simulink model "q_aero_2dof_pid_control"  (R2014a)
settings: Solver=ode1  StartTime=0.0  StopTime=inf  FixedStep=0.002  RelTol=1e-3
PreLoadFcn:
  | quanser_aero_pd_design;
values from neighbouring files (symbols this model uses):
  kp_p = tau*wn^2/K    [quanser_aero_pd_design.m]    (also in quanser_aero_pd_design_Ksp.m = (Jp*wn^2-Ksp)/Kpp)
  kp_y = tau*wn^2/K    [quanser_aero_pd_design.m]    (also in quanser_aero_pd_design_Ksp.m = Jy*wn^2/Kyy)
libraries: simulink_extras x4, quarc_library x3, quanser_aero x1
settings Model: SimulationMode=external  ExtModeTrigDuration=15000  Creator=MLevis  LastModifiedBy=MLevis
settings SolverCC: PositivePriorityOrder=on
settings DebuggingCC: MergeDetectMultiDrivingBlocksExec=error
settings RTWCC: SystemTargetFile=quarc_win64.tlc  TemplateMakefile=quarc_default_tmf  Description=QUARC Win64 Target  ProcessScript=quarc_win64_make_rtw_hook
settings GRTTargetCC: ParMdlRefBuildCompliant=off  CompOptLevelCompliant=off  CombineOutputUpdateFcns=off  MatFileLogging=off  CPPClassGenCompliant=off  GRTInterface=on  ExtMode=on  ExtModeMexFile=quarc_comm

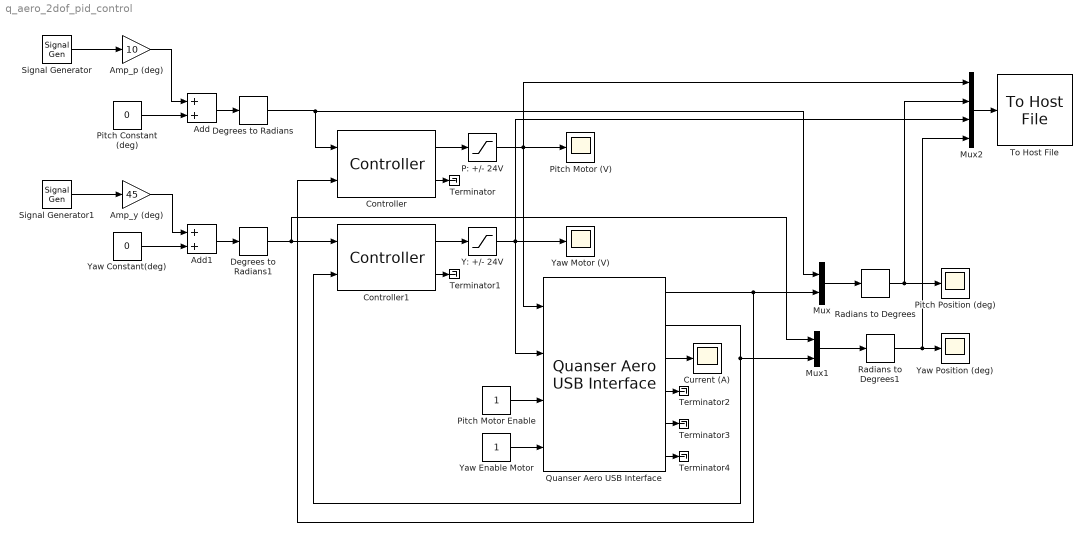
== system q_aero_2dof_pid_control ==
  Add : Sum
  Add1 : Sum
  Amp_p (deg) : Gain  Gain=10
  Amp_y (deg) : Gain  Gain=45
  Controller : quarc_library/Continuous/Controller  ctrl_type=Proportional-Integral-Velocity (PIV)  param_src=Specify via dialog  Kp=kp_p  Ki=0  Kd=0  Kv=kd_p  Ka=0  Wn=100
  Controller1 : quarc_library/Continuous/Controller  ctrl_type=Proportional-Integral-Velocity (PIV)  param_src=Specify via dialog  Kp=kp_y  Ki=0  Kd=0  Kv=kd_y  Ka=0  Wn=100
  Current (A) : Scope
      settings: TimeRange=5
  Degrees to Radians : simulink_extras/Transformations/Degrees to Radians
  Degrees to Radians1 : simulink_extras/Transformations/Degrees to Radians
  Mux : Mux  Inputs=2
  Mux1 : Mux  Inputs=2
  Mux2 : Mux
  P: +/- 24V : Saturate  UpperLimit=24  LowerLimit=-24
  Pitch Constant (deg) : Constant  Value=0
  Pitch Motor (V) : Scope
      settings: TimeRange=30  YMin=-30  YMax=30  SaveName=ScopeData2  MaxDataPoints=15000
  Pitch Motor Enable : Constant
  Pitch Position (deg) : Scope
      settings: TimeRange=30  YMin=-45  YMax=45  SaveName=ScopeData3  MaxDataPoints=15000
  Quanser Aero USB Interface : quanser_aero/Quanser Aero USB Interface
  Radians to Degrees : simulink_extras/Transformations/Radians to Degrees
  Radians to Degrees1 : simulink_extras/Transformations/Radians to Degrees
  Signal Generator : SignalGenerator  WaveForm=square  Frequency=0.1
  Signal Generator1 : SignalGenerator  WaveForm=square  Frequency=0.04
  Terminator{,1..4} (5 alike) : Terminator
  To Host File : quarc_library/Sinks/To Host/To Host File  file_name=aero_pid_rsp.mat  variable_name=pid_rsp  decimation=1  sample_time=-1  file_format=MAT-file v.4  options=No header or footer  append=off  final_file_name=aero_pid_rsp.mat
  Y: +/- 24V : Saturate  UpperLimit=24  LowerLimit=-24
  Yaw Constant(deg) : Constant  Value=0
  Yaw Enable Motor : Constant
  Yaw Motor (V) : Scope
      settings: TimeRange=30  YMin=-30  YMax=30  SaveName=ScopeData5  MaxDataPoints=15000
  Yaw Position (deg) : Scope
      settings: TimeRange=30  YMin=-100  YMax=100  SaveName=ScopeData4  MaxDataPoints=15000
  wires:
  Quanser Aero USB Interface/3 -> Current (A)/1
  Quanser Aero USB Interface/1 -> Controller/2, Mux/2
  Controller/1 -> P: +/- 24V/1
  Degrees to Radians/1 -> Mux/1, Controller/1
  Controller1/1 -> Y: +/- 24V/1
  Degrees to Radians1/1 -> Controller1/1, Mux1/1
  Quanser Aero USB Interface/2 -> Controller1/2, Mux1/2
  Controller/2 -> Terminator/1
  Controller1/2 -> Terminator1/1
  Signal Generator/1 -> Amp_p (deg)/1
  Pitch Constant (deg)/1 -> Add/2
  Add/1 -> Degrees to Radians/1
  Yaw Constant(deg)/1 -> Add1/2
  Amp_p (deg)/1 -> Add/1
  Signal Generator1/1 -> Amp_y (deg)/1
  Amp_y (deg)/1 -> Add1/1
  Add1/1 -> Degrees to Radians1/1
  Mux/1 -> Radians to Degrees/1
  Radians to Degrees/1 -> Mux2/2, Pitch Position (deg)/1
  Mux1/1 -> Radians to Degrees1/1
  Radians to Degrees1/1 -> Yaw Position (deg)/1, Mux2/4
  Pitch Motor Enable/1 -> Quanser Aero USB Interface/3
  Yaw Enable Motor/1 -> Quanser Aero USB Interface/4
  P: +/- 24V/1 -> Mux2/1, Quanser Aero USB Interface/1, Pitch Motor (V)/1
  Y: +/- 24V/1 -> Quanser Aero USB Interface/2, Mux2/3, Yaw Motor (V)/1
  Quanser Aero USB Interface/4 -> Terminator2/1
  Quanser Aero USB Interface/5 -> Terminator3/1
  Quanser Aero USB Interface/6 -> Terminator4/1
  Mux2/1 -> To Host File/1
